simulink model "posModel2"  (R2021b)
settings: Solver=ode5  StartTime=0.0  StopTime=131.071  FixedStep=dt  RelTol=1e-3
values from neighbouring files (symbols this model uses):
  Bm = bm * gearRatio * gearRatio    (= 2.601)    [posInit1.m]    (also in posInit2.m; posInit3.m)
  Jm = jm * gearRatio * gearRatio    (= 0.023968215)    [posInit1.m]    (also in posInit2.m; posInit3.m)
  kd = 1    [posInit1.m]    (also in posInit2.m; posInit3.m)
  kp = 50    [posInit1.m]    (also in posInit2.m; posInit3.m = 80)
  q0 = 0    [posInit1.m]    (also in posInit2.m; posInit3.m)
  qdot0 = 0    [posInit1.m]    (also in posInit2.m; posInit3.m)
libraries: simulink x3
settings Model: Creator=86135  LastModifiedBy=86135

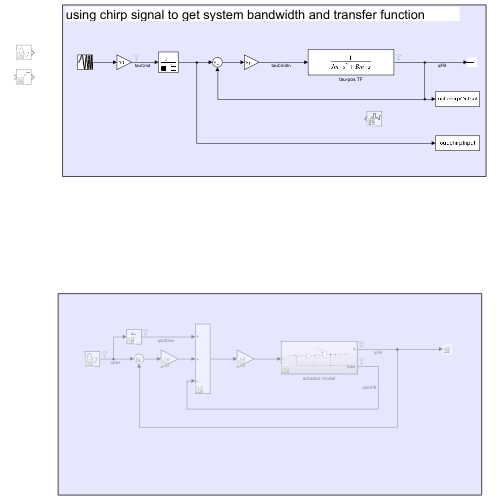
[thumbnail: Simulink's stored preview of the top-level diagram]
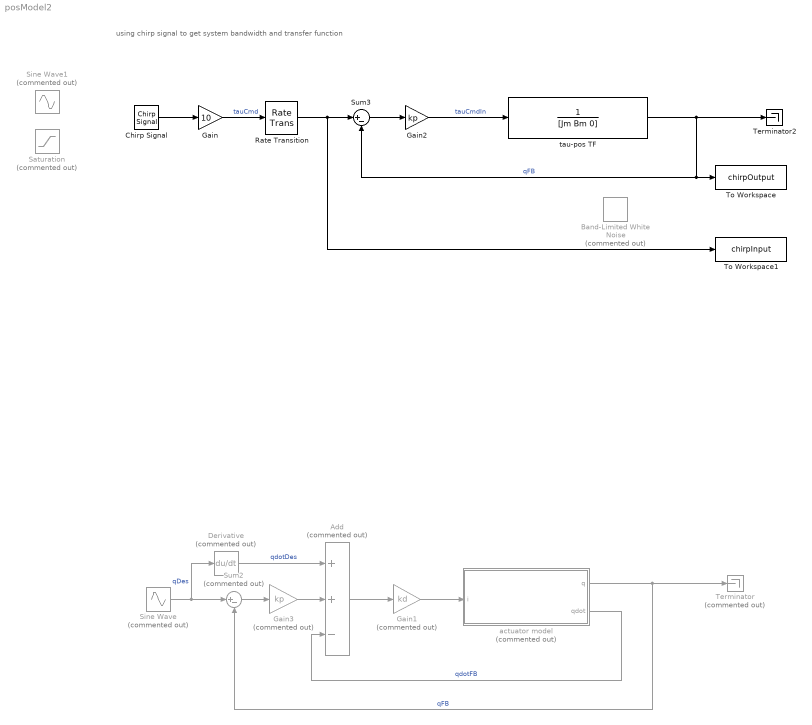
== system posModel2 ==
  note: using chirp signal to get system bandwidth and transfer function
  Add : Sum  Commented=on  Inputs=++-
  Band-Limited White Noise : simulink/Sources/Band-Limited White Noise  Commented=on  Cov=[0.00001]  Ts=0.001  seed=[11341]
  Chirp Signal : simulink/Sources/Chirp Signal  f1=f0  T=131.071  f2=f1
  Derivative : Derivative  Commented=on
  Gain : Gain  Gain=10
  Gain1 : Gain  Commented=on  Gain=kd
  Gain2 : Gain  Gain=kp
  Gain3 : Gain  Commented=on  Gain=kp
  Rate Transition : RateTransition  OutPortSampleTime=0.001
  Saturation : Saturate  Commented=on  UpperLimit=100  LowerLimit=-100
  Sine Wave : Sin  Commented=on  Frequency=2  SampleTime=0
  Sine Wave1 : Sin  Commented=on  Frequency=23  SampleTime=0
  Sum2 : Sum  Commented=on  Inputs=|+-
  Sum3 : Sum  Inputs=|+-
  Terminator : Terminator  Commented=on
  Terminator2 : Terminator
  To Workspace : ToWorkspace  VariableName=chirpOutput  SaveFormat=Timeseries  SampleTime=-1
  To Workspace1 : ToWorkspace  VariableName=chirpInput  SaveFormat=Timeseries  SampleTime=-1
  actuator model : Subsystem  Commented=on
  tau-pos TF : TransferFcn  Denominator=[Jm Bm 0]
  wires:
  actuator model/1(q) -> Terminator/1, Sum2/2  "qFB"
  Sum2/1 -> Gain3/1
  Sine Wave/1 -> Sum2/1, Derivative/1  "qDes"
  actuator model/2(qdot) -> Add/3  "qdotFB"
  Gain3/1 -> Add/2
  Gain1/1 -> actuator model/1(i)
  Add/1 -> Gain1/1
  Derivative/1 -> Add/1  "qdotDes"
  Sum3/1 -> Gain2/1
  Rate Transition/1 -> Sum3/1, To Workspace1/1
  Chirp Signal/1 -> Gain/1
  Gain/1 -> Rate Transition/1  "tauCmd"
  tau-pos TF/1 -> Sum3/2, To Workspace/1, Terminator2/1  "qFB"
  Gain2/1 -> tau-pos TF/1  "tauCmdIn"

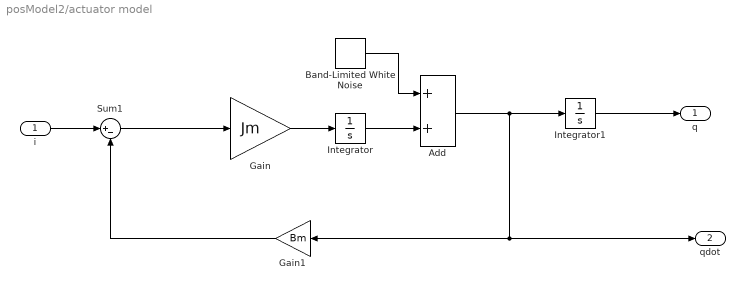
== system posModel2/actuator model ==
  i : Inport
  Add : Sum
  Band-Limited White Noise : simulink/Sources/Band-Limited White Noise  Cov=[0.00001]  Ts=0.001  seed=[16666]
  Gain : Gain  Gain=Jm
  Gain1 : Gain  Gain=Bm
  Integrator : Integrator  InitialCondition=qdot0
  Integrator1 : Integrator  InitialCondition=q0
  Sum1 : Sum  Inputs=|+-
  q : Outport
  qdot : Outport  Port=2
  wires:
  i/1 -> Sum1/1
  Sum1/1 -> Gain/1
  Gain1/1 -> Sum1/2
  Gain/1 -> Integrator/1
  Integrator1/1 -> q/1
  Integrator/1 -> Add/2
  Add/1 -> Gain1/1, qdot/1, Integrator1/1
  Band-Limited White Noise/1 -> Add/1
